simulink model "leuschner_spectrometer"  (Simulink 6.2)
settings: Solver=ode45  StartTime=0.0  StopTime=10  RelTol=1e-3
undefined symbols (not defined in the file): MaxCoeffNum
libraries: xbsIndex_r3 x225, fft_library x17, xps_library x14, delay_lib x4, casper_library x3, simulink x1, pfb_library x1
(part 1 of 2)
settings Model: LastModifiedBy=siemion
settings DebuggingCC: SolverPrmCheckMsg=warning

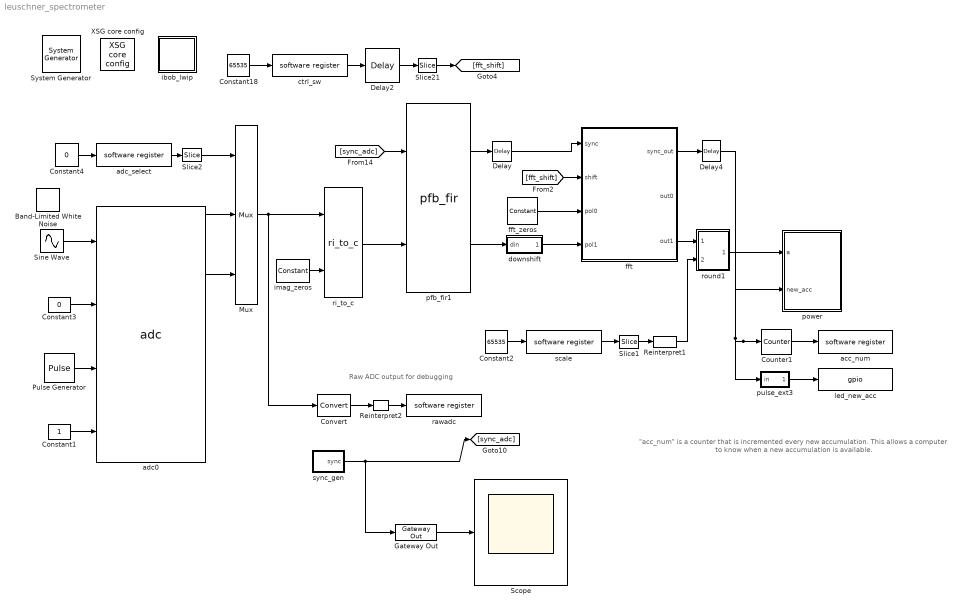
== system leuschner_spectrometer ==
  note: Raw ADC output for debugging
  note: "acc_num" is a counter that is
      | incremented every new accumulation.
      | This allows a computer to know when
      | a new accumulation is available.
  " System Generator" : xbsIndex_r3/ System Generator  Tag=genX  xilinxfamily=Virtex2P  part=xc2vp50  speed=-7  package=ff1152  synthesis_tool=XST  directory=./heilesspec_two_inp/sysgen  testbench=off  simulink_period=1  sysclk_period=41.6667  incr_netlist=off  trim_vbits=Everywhere in SubSystem  dbl_ovrd=According to Block Masks  core_generation=According to Block Masks  run_coregen=off  deprecated_control=off  eval_field=0
      settings: AttributesFormatString=System\nGenerator
  Band-Limited White Noise : simulink/Sources/Band-Limited White Noise  Cov=[0.1]  Ts=0.1  seed=[23341]
  Constant1 : Constant
  Constant18 : Constant  Value=65535
  Constant2 : Constant  Value=65535
  Constant3 : Constant  Value=0
  Constant4 : Constant  Value=0
  Convert : xbsIndex_r3/Convert  arith_type="Signed  (2's comp)"  n_bits=32  bin_pt=7  quantization=Truncate  overflow=Wrap  latency=0  explicit_period=off  period=1  dbl_ovrd=off  show_param=off  inserted_by_tool=off  pipeline=off
      settings: xl_area=[0, 0, 0, 0, 0, 0, 0]
  Counter1 : xbsIndex_r3/Counter  cnt_type=Free Running  n_bits=32  bin_pt=0  arith_type=Unsigned  start_count=0  cnt_to=Inf  cnt_by_val=1  operation=Up  explicit_period=off  period=1  load_pin=off  rst=off  en=on  dbl_ovrd=off  show_param=off  use_rpm=on  gen_core=off
      settings: xl_area=[0, 0, 0, 0, 0, 0, 0]
  Delay : xbsIndex_r3/Delay  latency=2  reg_retiming=off  explicit_period=off  period=1  en=off  accept_only_valid=off  init_zero=on  dbl_ovrd=off  show_param=off
      settings: xl_area=[0, 0, 0, 0, 0, 0, 0]
  Delay2 : xbsIndex_r3/Delay  latency=1  reg_retiming=off  explicit_period=off  period=1  en=off  accept_only_valid=off  init_zero=on  dbl_ovrd=off  show_param=off
      settings: xl_area=[0, 0, 0, 0, 0, 0, 0]
  Delay4 : xbsIndex_r3/Delay  latency=4  reg_retiming=off  explicit_period=off  period=1  en=off  accept_only_valid=off  init_zero=on  dbl_ovrd=off  show_param=off
      settings: xl_area=[0, 0, 0, 0, 0, 0, 0]
  Gateway Out : xbsIndex_r3/Gateway Out  output_type=Double  nbits=8  bin_pt=6  arith_type=Boolean  quantization=Truncate  overflow=Wrap  hdl_port=on  timing_constraint=None  locs_specified=off  LOCs={}  needs_fixed_name=off  show_param=off
      settings: xl_area=[0, 0, 0, 0, 0, 0, 0]
  Mux : xbsIndex_r3/Mux  inputs=2  precision=Full  arith_type="Signed  (2's comp)"  n_bits=8  bin_pt=2  quantization=Truncate  overflow=Wrap  latency=0  explicit_period=off  period=1  en=off  dbl_ovrd=off  show_param=off  mux_type=off  use_rpm=off  gen_core=off
      settings: xl_area=[0, 0, 0, 0, 0, 0, 0]
  Pulse Generator : DiscretePulseGenerator  Period=2^9
  Reinterpret1 : xbsIndex_r3/Reinterpret  force_arith_type=on  arith_type=Unsigned  force_bin_pt=on  bin_pt=3  force_valid=on
  Reinterpret2 : xbsIndex_r3/Reinterpret  force_arith_type=on  arith_type=Unsigned  force_bin_pt=on  bin_pt=0  force_valid=on
  Scope : Scope
      settings: YMin=-1  YMax=1
  Sine Wave : Sin  SineType=Sample based  Amplitude=0.2  Frequency=2*pi*0.5  Samples=8  SampleTime=1
  Slice1 : xbsIndex_r3/Slice  mode=Lower Bit Location + Width  nbits=18  bit1=0  base1=MSB of Input  bit0=0  base0=LSB of Input  boolean_output=off  explicit_period=off  period=1  dbl_ovrd=off
  Slice2 : xbsIndex_r3/Slice  mode=Lower Bit Location + Width  nbits=1  bit1=0  base1=MSB of Input  bit0=0  base0=LSB of Input  boolean_output=on  explicit_period=off  period=1  dbl_ovrd=off
  Slice21 : xbsIndex_r3/Slice  mode=Lower Bit Location + Width  nbits=16  bit1=0  base1=MSB of Input  bit0=0  base0=LSB of Input  boolean_output=off  explicit_period=off  period=1  dbl_ovrd=off
  XSG core config : xps_library/XSG core config  Tag=xps:xsg  hw_sys=iBOB  ibob_linux=off  clk_src=adc0_clk  gpio_clk_io_group=iBOB:sma  gpio_clk_bit_index=0  clk_rate=24  sample_period=1  synthesis_tool=XST  mpc_type=powerpc405
  acc_num : xps_library/software register  Tag=xps:sw_reg  io_dir=To Processor  arith_type=Unsigned  bitwidth=32  bin_pt=0  sample_period=1  gw_name=heilesspec_two_inp_acc_num_user_data_in
  adc0 : xps_library/adc  Tag=xps:adc  adc_brd=iBOB:adc0  adc_clk_rate=96  adc_interleave=off  sample_period=1
  adc_select : xps_library/software register  Tag=xps:sw_reg  io_dir=From Processor  arith_type=Unsigned  bitwidth=32  bin_pt=0  sample_period=1  gw_name=heilesspec_two_inp_adc_select_user_data_out
  ctrl_sw : xps_library/software register  Tag=xps:sw_reg  io_dir=From Processor  arith_type=Unsigned  bitwidth=32  bin_pt=0  sample_period=1  gw_name=heilesspec_two_inp_ctrl_sw_user_data_out
  downshift : Subsystem
  fft : Subsystem  AncestorBlock=fft_library/fft  mask{FFTSize=14, BitWidth=18, n_inputs=0, quantization=Truncate, overflow=Wrap, add_latency=2, mult_latency=4, bram_latency=1}
      mask prompts: FFTSize "Size of FFT: (2^?)"; BitWidth "Bit Width"; n_inputs "Number of Simultaneous Inputs: (2^?)"; quantization "Quantization Behavior"; overflow "Overflow Behavior"; add_latency "Add Latency"; mult_latency "Mult Latency"; bram_latency "BRAM Latency"
      mask init:
      | fft_mask;
      mask StyleString: edit,edit,edit,popup(Truncate|Round  (unbiased: +/- Inf)|Round  (unbiased: Even Values)),popup(Wrap|Saturate|Error),edit,edit,edit
  fft_zeros : xbsIndex_r3/Constant  const=0  equ=P=C  arith_type=Unsigned  n_bits=36  bin_pt=0  opselect=C  inp2=PCIN>>17  opr=+  inp1=P  carry=CIN  iostate=0  explicit_period=on  period=1  dbl_ovrd=off
  ibob_lwip : Subsystem  AncestorBlock=xps_library/ibob_lwip
      mask Type: ibobethlite
      mask Description: Attaches SRAM0 to the PLB bus and adds LWIP support.
      mask Display: fprintf('IBOB\nLWIP');
  imag_zeros : xbsIndex_r3/Constant  const=0  equ=P=C  arith_type="Signed  (2's comp)"  n_bits=8  bin_pt=7  opselect=C  inp2=PCIN>>17  opr=+  inp1=P  carry=CIN  iostate=0  explicit_period=on  period=1  dbl_ovrd=off
  led_new_acc : xps_library/gpio  Tag=xps:gpio  io_group=iBOB:led  io_dir=out  arith_type=Boolean  bitwidth=1  bin_pt=0  bit_index=5  sample_period=1  use_single_ended=off  use_ddr=off  reg_iob=on  reg_clk_phase=0  termination=None
  pfb_fir1 : pfb_library/pfb_fir  PFBSize=14  TotalTaps=2  WindowType=hamming  n_inputs=0  MakeBiplex=off  BitWidthIn=8  BitWidthOut=18  CoeffBitWidth=8  CoeffDistMem=on  add_latency=2  mult_latency=3  bram_latency=2  quantization="Round  (unbiased: +/- Inf)"  fwidth=1
      link override pol1_in1_first_tap/sync_delay/Constant: equ=P=C
      link override pol1_in1_first_tap/sync_delay/Constant1: equ=P=C
      link override pol1_in1_first_tap/sync_delay/Constant2: equ=P=C
      link override pol1_in1_first_tap/sync_delay/Constant3: equ=P=C
  power : Subsystem
  pulse_ext3 : Subsystem  mask{pulse_len=2^23}
      mask prompts: pulse_len "Length of Pulse"
      mask init:
      | bits = ceil(log2(pulse_len+1));
  rawadc : xps_library/software register  Tag=xps:sw_reg  io_dir=To Processor  arith_type=Unsigned  bitwidth=32  bin_pt=0  sample_period=1  gw_name=heilesspec_two_inp_rawadc_user_data_in
  ri_to_c : fft_library/ri_to_c  likes_cookies=on
  round1 : Subsystem
  scale : xps_library/software register  Tag=xps:sw_reg  io_dir=From Processor  arith_type=Unsigned  bitwidth=32  bin_pt=0  sample_period=1  gw_name=heilesspec_two_inp_scale_user_data_out
  sync_gen : Subsystem
  wires:
  Pulse Generator/1 -> adc0/3
  Constant1/1 -> adc0/4
  pfb_fir1/1 -> Delay/1
  sync_gen/1(sync) -> Gateway Out/1, [sync_adc]
  Constant18/1 -> ctrl_sw/1
  ctrl_sw/1 -> Delay2/1
  Slice21/1 -> [fft_shift]
  [sync_adc] -> pfb_fir1/1
  [fft_shift] -> fft/2(shift)
  fft/1(sync_out) -> Delay4/1
  pulse_ext3/1(out) -> led_new_acc/1
  Counter1/1 -> acc_num/1
  Delay2/1 -> Slice21/1
  pfb_fir1/2 -> downshift/1(din)
  Delay/1 -> fft/1(sync)
  Gateway Out/1 -> Scope/1
  Constant3/1 -> adc0/2
  imag_zeros/1 -> ri_to_c/2
  ri_to_c/1 -> pfb_fir1/2
  downshift/1(dout) -> fft/4(pol1)
  Sine Wave/1 -> adc0/1
  fft_zeros/1 -> fft/3(pol0)
  Reinterpret1/1 -> round1/2(scale)
  Delay4/1 -> power/2(new_acc), pulse_ext3/1(in), Counter1/1
  fft/3(out1) -> round1/1(din)
  Constant2/1 -> scale/1
  scale/1 -> Slice1/1
  Slice1/1 -> Reinterpret1/1
  adc0/1 -> Mux/2
  adc0/5 -> Mux/3
  Slice2/1 -> Mux/1
  adc_select/1 -> Slice2/1
  Convert/1 -> Reinterpret2/1
  Mux/1 -> Convert/1, ri_to_c/1
  Reinterpret2/1 -> rawadc/1
  Constant4/1 -> adc_select/1
  round1/1(dout) -> power/1(a)

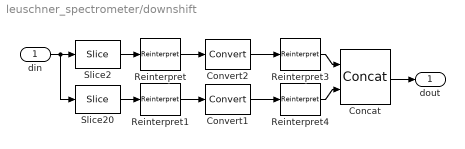
== system leuschner_spectrometer/downshift ==
  din : Inport  Port=1  LatchInput=off
  Concat : xbsIndex_r3/Concat  num_inputs=2  explicit_period=off  period=1  dbl_ovrd=off
  Convert1 : xbsIndex_r3/Convert  arith_type="Signed  (2's comp)"  n_bits=18  bin_pt=15  quantization="Round  (unbiased: Even Values)"  overflow=Wrap  latency=2  explicit_period=off  period=1  dbl_ovrd=off  show_param=off  inserted_by_tool=off  pipeline=off
      settings: xl_area=[0, 0, 0, 0, 0, 0, 0]
  Convert2 : xbsIndex_r3/Convert  arith_type="Signed  (2's comp)"  n_bits=18  bin_pt=15  quantization="Round  (unbiased: Even Values)"  overflow=Wrap  latency=2  explicit_period=off  period=1  dbl_ovrd=off  show_param=off  inserted_by_tool=off  pipeline=off
      settings: xl_area=[0, 0, 0, 0, 0, 0, 0]
  Reinterpret : xbsIndex_r3/Reinterpret  force_arith_type=on  arith_type="Signed  (2's comp)"  force_bin_pt=on  bin_pt=17  force_valid=on
  Reinterpret1 : xbsIndex_r3/Reinterpret  force_arith_type=on  arith_type="Signed  (2's comp)"  force_bin_pt=on  bin_pt=17  force_valid=on
  Reinterpret3 : xbsIndex_r3/Reinterpret  force_arith_type=on  arith_type=Unsigned  force_bin_pt=on  bin_pt=0  force_valid=on
  Reinterpret4 : xbsIndex_r3/Reinterpret  force_arith_type=on  arith_type=Unsigned  force_bin_pt=on  bin_pt=0  force_valid=on
  Slice2 : xbsIndex_r3/Slice  mode=Upper Bit Location + Width  nbits=18  bit1=0  base1=MSB of Input  bit0=0  base0=LSB of Input  boolean_output=off  explicit_period=off  period=1  dbl_ovrd=off
  Slice20 : xbsIndex_r3/Slice  mode=Lower Bit Location + Width  nbits=18  bit1=0  base1=MSB of Input  bit0=0  base0=LSB of Input  boolean_output=off  explicit_period=off  period=1  dbl_ovrd=off
  dout : Outport
  wires:
  Slice2/1 -> Reinterpret/1
  Slice20/1 -> Reinterpret1/1
  din/1 -> Slice2/1, Slice20/1
  Reinterpret3/1 -> Concat/1
  Reinterpret4/1 -> Concat/2
  Concat/1 -> dout/1
  Reinterpret/1 -> Convert2/1
  Reinterpret1/1 -> Convert1/1
  Convert2/1 -> Reinterpret3/1
  Convert1/1 -> Reinterpret4/1

== system leuschner_spectrometer/fft ==
  sync : Inport  Port=1  LatchInput=off
  shift : Inport  Port=2  LatchInput=off
  pol0 : Inport  Port=3  LatchInput=off
  pol1 : Inport  Port=4  LatchInput=off
  fft_biplex0 : Subsystem  AncestorBlock=fft_library/fft_biplex  mask(fft_biplex){FFTSize=FFTSize-n_inputs, BitWidth=BitWidth, quantization=Truncate, overflow=Wrap, add_latency=add_latency, mult_latency=mult_latency, bram_latency=bram_latency}
      mask prompts: FFTSize "Size of FFT: (2^? pnts)"; BitWidth "Bitwidth: (Max Efficiency at 18 bits)"; quantization "Quantization Behavior"; overflow "Overflow Behavior"; add_latency "Add Latency"; mult_latency "Mult Latency"; bram_latency "BRAM Latency"
      mask init:
      | cursys = gcb;
      | disp(cursys);
      | biplex_core = [cursys,'/biplex_core'];
      | if ~strcmp(get_param(biplex_core, 'quantization'), quantization),
      |     set_param(biplex_core, 'quantization', quantization);
      | end
      | if ~strcmp(get_param(biplex_core, 'overflow'), overflow),
      |     set_param(biplex_core, 'overflow', overflow);
      | end
      mask StyleString: edit,edit,popup(Truncate|Round  (unbiased: +/- Inf)|Round  (unbiased: Even Values)),popup(Wrap|Saturate|Error),edit,edit,edit
  sync_out : Outport
  out0 : Outport  Port=2
  out1 : Outport  Port=3

== system leuschner_spectrometer/ibob_lwip ==
  Constant : Constant  Value=0
  Terminator : Terminator
  ethlite : Subsystem  Tag=xps:ethlite
      mask Type: ethlite
      mask Description: Instantiates an opb_ethernetlite core into the design.
      mask Display: fprintf('ETHLITE');
  lwip : Subsystem  Tag=xps:lwip
      mask Type: lwip
      mask Description: Attaches SRAM0 to the PLB bus and adds LWIP support.
      mask Display: fprintf('LWIP');
  macbits : xps_library/software register  Tag=xps:sw_reg  io_dir=To Processor  arith_type=Unsigned  bitwidth=32  bin_pt=0  sample_period=1  gw_name=heilesspec_two_inp_ibob_lwip_macbits_user_data_in
  machdr : xps_library/gpio  Tag=xps:gpio  io_group=iBOB:gpio2  io_dir=in  arith_type=Unsigned  bitwidth=20  bin_pt=0  bit_index=[0:19]  sample_period=1  use_single_ended=off  use_ddr=off  reg_iob=off  reg_clk_phase=0  termination=Pullup
  wires:
  Constant/1 -> machdr/1
  macbits/1 -> Terminator/1
  machdr/1 -> macbits/1

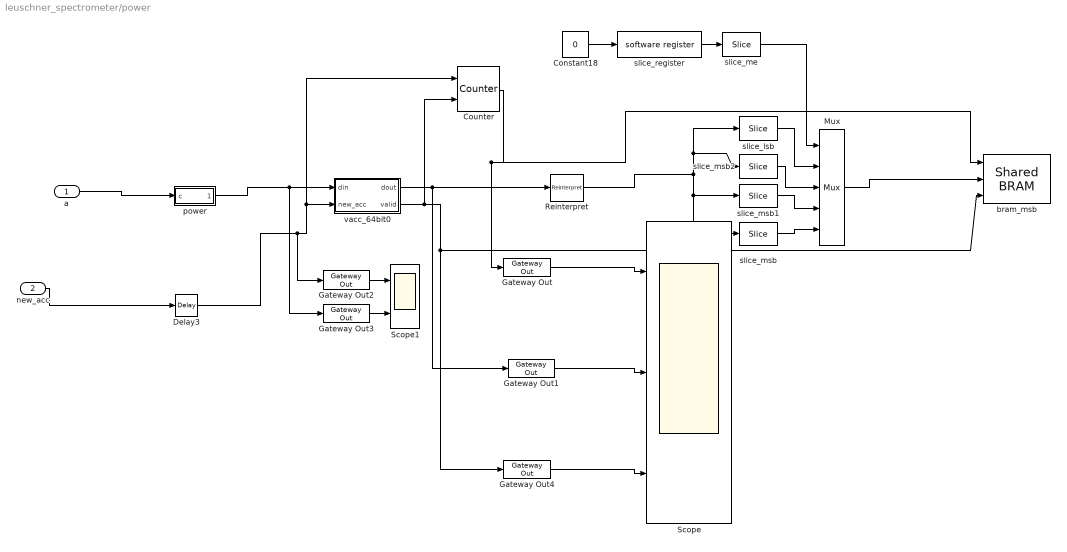
== system leuschner_spectrometer/power ==
  a : Inport  Port=1  LatchInput=off
  new_acc : Inport  Port=2  LatchInput=off
  Constant18 : Constant  Value=0
  Counter : xbsIndex_r3/Counter  cnt_type=Free Running  n_bits=13  bin_pt=0  arith_type=Unsigned  start_count=0  cnt_to=Inf  cnt_by_val=1  operation=Up  explicit_period=off  period=1  load_pin=off  rst=on  en=on  dbl_ovrd=off  show_param=off  use_rpm=on  gen_core=off
      settings: xl_area=[0, 0, 0, 0, 0, 0, 0]
  Delay3 : xbsIndex_r3/Delay  latency=5  reg_retiming=off  explicit_period=off  period=1  en=off  accept_only_valid=off  init_zero=on  dbl_ovrd=off  show_param=off
      settings: xl_area=[0, 0, 0, 0, 0, 0, 0]
  Gateway Out{,1..4} (5 alike) : xbsIndex_r3/Gateway Out  output_type=Double  nbits=8  bin_pt=6  arith_type=Boolean  quantization=Truncate  overflow=Wrap  hdl_port=on  timing_constraint=None  locs_specified=off  LOCs={}  needs_fixed_name=off  show_param=off
      settings: xl_area=[0, 0, 0, 0, 0, 0, 0]
  Mux : xbsIndex_r3/Mux  inputs=4  precision=Full  arith_type="Signed  (2's comp)"  n_bits=8  bin_pt=2  quantization=Truncate  overflow=Wrap  latency=0  explicit_period=off  period=1  en=off  dbl_ovrd=off  show_param=off  mux_type=off  use_rpm=off  gen_core=off
      settings: xl_area=[0, 0, 0, 0, 0, 0, 0]
  Reinterpret : xbsIndex_r3/Reinterpret  force_arith_type=on  arith_type="Signed  (2's comp)"  force_bin_pt=on  bin_pt=0  force_valid=on
  Scope : Scope  NumInputPorts=3
      settings: YMin=0~0~0  YMax=2100~0.00095~1
  Scope1 : Scope  NumInputPorts=2
      settings: YMin=-1~0  YMax=1~0.00045  SaveName=ScopeData2
  bram_msb : xps_library/Shared BRAM  Tag=xps:bram  arith_type=Unsigned  addr_width=13  data_width=32  data_bin_pt=0  init_vals=[1:2^11]  sample_rate=1
  power : Subsystem  AncestorBlock=casper_library/Misc/power  mask{BitWidth=18}
      mask prompts: BitWidth "Bit Width"
  slice_lsb : xbsIndex_r3/Slice  mode=Lower Bit Location + Width  nbits=32  bit1=0  base1=LSB of Input  bit0=0  base0=LSB of Input  boolean_output=off  explicit_period=off  period=1  dbl_ovrd=off
  slice_me : xbsIndex_r3/Slice  mode=Lower Bit Location + Width  nbits=2  bit1=0  base1=LSB of Input  bit0=0  base0=LSB of Input  boolean_output=off  explicit_period=off  period=1  dbl_ovrd=off
  slice_msb : xbsIndex_r3/Slice  mode=Lower Bit Location + Width  nbits=32  bit1=0  base1=LSB of Input  bit0=32  base0=LSB of Input  boolean_output=off  explicit_period=off  period=1  dbl_ovrd=off
  slice_msb1 : xbsIndex_r3/Slice  mode=Lower Bit Location + Width  nbits=32  bit1=0  base1=LSB of Input  bit0=16  base0=LSB of Input  boolean_output=off  explicit_period=off  period=1  dbl_ovrd=off
  slice_msb2 : xbsIndex_r3/Slice  mode=Lower Bit Location + Width  nbits=32  bit1=0  base1=LSB of Input  bit0=8  base0=LSB of Input  boolean_output=off  explicit_period=off  period=1  dbl_ovrd=off
  slice_register : xps_library/software register  Tag=xps:sw_reg  io_dir=From Processor  arith_type=Unsigned  bitwidth=32  bin_pt=0  sample_period=1  gw_name=heilesspec_two_inp_power_slice_register_user_data_out
  vacc_64bit0 : Subsystem
  wires:
  new_acc/1 -> Delay3/1
  power/1(power) -> vacc_64bit0/1(din), Gateway Out3/1
  vacc_64bit0/1(dout) -> Reinterpret/1, Gateway Out1/1
  Delay3/1 -> Counter/1, vacc_64bit0/2(new_acc), Gateway Out2/1
  vacc_64bit0/2(valid) -> Counter/2, bram_msb/3, Gateway Out4/1
  Counter/1 -> Gateway Out/1, bram_msb/1
  Gateway Out/1 -> Scope/1
  Gateway Out1/1 -> Scope/2
  Gateway Out2/1 -> Scope1/1
  Gateway Out3/1 -> Scope1/2
  a/1 -> power/1(c)
  Reinterpret/1 -> slice_lsb/1, slice_msb2/1, slice_msb/1, slice_msb1/1
  Gateway Out4/1 -> Scope/3
  slice_lsb/1 -> Mux/2
  Mux/1 -> bram_msb/2
  slice_register/1 -> slice_me/1
  Constant18/1 -> slice_register/1
  slice_me/1 -> Mux/1
  slice_msb2/1 -> Mux/3
  slice_msb1/1 -> Mux/4
  slice_msb/1 -> Mux/5

== system leuschner_spectrometer/pulse_ext3 ==
  in : Inport  Port=1  LatchInput=off
  Constant5 : xbsIndex_r3/Constant  const=pulse_len  equ=P=C  arith_type=Unsigned  n_bits=bits  bin_pt=0  opselect=C  inp2=PCIN>>17  opr=+  inp1=P  carry=CIN  iostate=0  explicit_period=off  period=1  dbl_ovrd=off
  Counter3 : xbsIndex_r3/Counter  cnt_type=Free Running  n_bits=bits  bin_pt=0  arith_type=Unsigned  start_count=0  cnt_to=1023  cnt_by_val=1  operation=Up  explicit_period=on  period=1  load_pin=off  rst=on  en=on  dbl_ovrd=off  show_param=off  use_rpm=on  gen_core=off
      settings: xl_area=[0, 0, 0, 0, 0, 0, 0]
  Relational5 : xbsIndex_r3/Relational  mode=a!=b  latency=0  explicit_period=off  period=1  en=off  dbl_ovrd=off  show_param=off
      settings: xl_area=[0, 0, 0, 0, 0, 0, 0]
  posedge : Subsystem  Tag=Rising Edge Detector
  out : Outport
  wires:
  Counter3/1 -> Relational5/1
  Constant5/1 -> Relational5/2
  Relational5/1 -> Counter3/2, out/1
  in/1 -> posedge/1(In)
  posedge/1(Out) -> Counter3/1

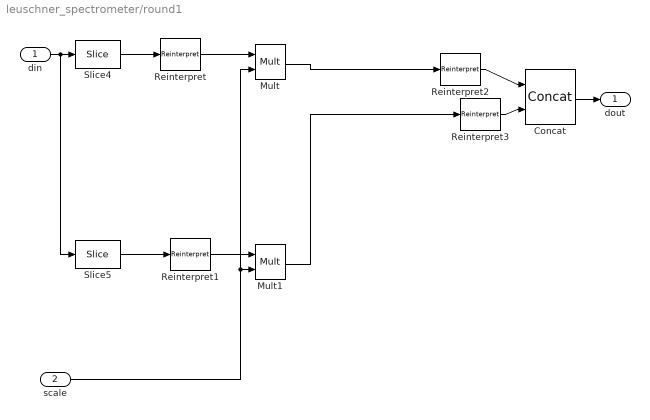
== system leuschner_spectrometer/round1 ==
  din : Inport  Port=1  LatchInput=off
  scale : Inport  Port=2  LatchInput=off
  Concat : xbsIndex_r3/Concat  num_inputs=2  explicit_period=off  period=1  dbl_ovrd=off
  Mult : xbsIndex_r3/Mult  precision=User Defined  arith_type="Signed  (2's comp)"  n_bits=18  bin_pt=17  quantization=Truncate  overflow=Saturate  latency=4  explicit_period=off  period=1  en=off  dbl_ovrd=off  show_param=on  mult_type=Parallel  oversample=2  use_embedded=on  pipeline=on  use_rpm=on  placement_style=Rectangular Shape  gen_core=off
      settings: xl_area=[0, 0, 0, 0, 0, 0, 0]
  Mult1 : xbsIndex_r3/Mult  precision=User Defined  arith_type="Signed  (2's comp)"  n_bits=18  bin_pt=17  quantization=Truncate  overflow=Saturate  latency=4  explicit_period=off  period=1  en=off  dbl_ovrd=off  show_param=on  mult_type=Parallel  oversample=2  use_embedded=on  pipeline=on  use_rpm=on  placement_style=Rectangular Shape  gen_core=off
      settings: xl_area=[0, 0, 0, 0, 0, 0, 0]
  Reinterpret : xbsIndex_r3/Reinterpret  force_arith_type=on  arith_type="Signed  (2's comp)"  force_bin_pt=on  bin_pt=17  force_valid=on
  Reinterpret1 : xbsIndex_r3/Reinterpret  force_arith_type=on  arith_type="Signed  (2's comp)"  force_bin_pt=on  bin_pt=17  force_valid=on
  Reinterpret2 : xbsIndex_r3/Reinterpret  force_arith_type=on  arith_type=Unsigned  force_bin_pt=on  bin_pt=0  force_valid=on
  Reinterpret3 : xbsIndex_r3/Reinterpret  force_arith_type=on  arith_type=Unsigned  force_bin_pt=on  bin_pt=0  force_valid=on
  Slice4 : xbsIndex_r3/Slice  mode=Upper Bit Location + Width  nbits=18  bit1=0  base1=MSB of Input  bit0=0  base0=LSB of Input  boolean_output=off  explicit_period=off  period=1  dbl_ovrd=off
  Slice5 : xbsIndex_r3/Slice  mode=Lower Bit Location + Width  nbits=18  bit1=0  base1=MSB of Input  bit0=0  base0=LSB of Input  boolean_output=off  explicit_period=off  period=1  dbl_ovrd=off
  dout : Outport
  wires:
  Slice4/1 -> Reinterpret/1
  Reinterpret2/1 -> Concat/1
  Slice5/1 -> Reinterpret1/1
  Reinterpret3/1 -> Concat/2
  din/1 -> Slice4/1, Slice5/1
  Concat/1 -> dout/1
  Reinterpret1/1 -> Mult1/1
  Reinterpret/1 -> Mult/1
  scale/1 -> Mult1/2, Mult/2
  Mult/1 -> Reinterpret2/1
  Mult1/1 -> Reinterpret3/1

== system leuschner_spectrometer/sync_gen ==
  note: NOTE: Outputs sync pulse immediately on RST
      | (i.e. when RST goes high, SYNC goes high, and the sync counter is reset)
  note: PERIOD must be the period you want, sub 2.
      | e.g. If you want 2048, enter 2046
  Constant : Constant  Value=2^12 * 8
  Convert : xbsIndex_r3/Convert  arith_type=Boolean  n_bits=8  bin_pt=6  quantization=Truncate  overflow=Wrap  latency=1  explicit_period=off  period=1  dbl_ovrd=off  show_param=off  inserted_by_tool=off  pipeline=off
      settings: xl_area=[0, 0, 0, 0, 0, 0, 0]
  Counter1 : xbsIndex_r3/Counter  cnt_type=Free Running  n_bits=32  bin_pt=0  arith_type=Unsigned  start_count=1  cnt_to=Inf  cnt_by_val=1  operation=Up  explicit_period=on  period=1  load_pin=off  rst=on  en=off  dbl_ovrd=off  show_param=off  use_rpm=on  gen_core=off
      settings: xl_area=[0, 0, 0, 0, 0, 0, 0]
  Relational : xbsIndex_r3/Relational  mode=a>=b  latency=1  explicit_period=off  period=1  en=off  dbl_ovrd=off  show_param=off
      settings: xl_area=[0, 0, 0, 0, 0, 0, 0]
  period : xps_library/software register  Tag=xps:sw_reg  io_dir=From Processor  arith_type=Unsigned  bitwidth=32  bin_pt=0  sample_period=1  gw_name=heilesspec_two_inp_sync_gen_period_user_data_out
  sync : Outport
  wires:
  Counter1/1 -> Relational/1
  Relational/1 -> Convert/1
  period/1 -> Relational/2
  Convert/1 -> Counter1/1, sync/1
  Constant/1 -> period/1

== system leuschner_spectrometer/fft/fft_biplex0 ==
  pol1 : Inport  Port=1  LatchInput=off
  pol2 : Inport  Port=2  LatchInput=off
  sync : Inport  Port=3  LatchInput=off
  shift : Inport  Port=4  LatchInput=off
  biplex_core : Subsystem  AncestorBlock=fft_library/biplex_core  mask{FFTSize=FFTSize, BitWidth=BitWidth, quantization=Truncate, overflow=Wrap, add_latency=add_latency, mult_latency=mult_latency, bram_latency=bram_latency}
      mask prompts: FFTSize "Size of FFT: (2^? pnts)"; BitWidth "Bitwidth: (Max Efficiency at 18 bits)"; quantization "Quantization Behavior"; overflow "Overflow Behavior"; add_latency "Add Latency"; mult_latency "Mult Latency"; bram_latency "BRAM Latency"
      mask init:
      | biplex_core_mask;
      mask StyleString: edit,edit,popup(Truncate|Round  (unbiased: +/- Inf)|Round  (unbiased: Even Values)),popup(Wrap|Saturate|Error),edit,edit,edit
  biplex_cplx_unscrambler : Subsystem
  pol1_out : Outport
  pol2_out : Outport  Port=2
  of : Outport  Port=3
  sync_out : Outport  Port=4
  wires:
  biplex_core/4(sync_out) -> biplex_cplx_unscrambler/3(sync)
  biplex_core/2(out2) -> biplex_cplx_unscrambler/2(odd)
  biplex_core/1(out1) -> biplex_cplx_unscrambler/1(even)
  biplex_core/3(of) -> of/1
  biplex_cplx_unscrambler/3(sync_out) -> sync_out/1
  biplex_cplx_unscrambler/2(pol2) -> pol2_out/1
  biplex_cplx_unscrambler/1(pol1) -> pol1_out/1
  shift/1 -> biplex_core/4(shift)
  sync/1 -> biplex_core/3(sync)
  pol2/1 -> biplex_core/2(pol2)
  pol1/1 -> biplex_core/1(pol1)

== system leuschner_spectrometer/ibob_lwip/ethlite ==

== system leuschner_spectrometer/ibob_lwip/lwip ==

== system leuschner_spectrometer/power/power ==
  c : Inport  Port=1  LatchInput=off
  c_to_ri : casper_library/Misc/c_to_ri  n_bits=BitWidth  bin_pt=BitWidth-1
      settings: AttributesFormatString=18_17 r/i
  imag_square : xbsIndex_r3/Mult  precision=Full  arith_type="Signed  (2's comp)"  n_bits=8  bin_pt=2  quantization=Truncate  overflow=Wrap  latency=3  explicit_period=off  period=1  en=off  dbl_ovrd=off  show_param=on  mult_type=Parallel  oversample=2  use_embedded=on  pipeline=on  use_rpm=on  placement_style=Rectangular Shape  gen_core=off
      settings: xl_area=[0, 0, 0, 0, 0, 0, 0]
  power_adder : xbsIndex_r3/AddSub  mode=Addition  precision=User Defined  arith_type=Unsigned  n_bits=BitWidth * 2  bin_pt=BitWidth * 2 - 1  quantization=Truncate  overflow=Wrap  latency=2  explicit_period=off  period=1  use_carryin=off  use_carryout=off  en=off  dbl_ovrd=off  show_param=off  use_core=on  pipeline=off  use_rpm=on  gen_core=off
      settings: xl_area=[0, 0, 0, 0, 0, 0, 0]
  real_square : xbsIndex_r3/Mult  precision=Full  arith_type="Signed  (2's comp)"  n_bits=8  bin_pt=2  quantization=Truncate  overflow=Wrap  latency=3  explicit_period=off  period=1  en=off  dbl_ovrd=off  show_param=on  mult_type=Parallel  oversample=2  use_embedded=on  pipeline=on  use_rpm=on  placement_style=Rectangular Shape  gen_core=off
      settings: xl_area=[0, 0, 0, 0, 0, 0, 0]
  power : Outport
  wires:
  power_adder/1 -> power/1
  imag_square/1 -> power_adder/2
  real_square/1 -> power_adder/1
  c/1 -> c_to_ri/1
  c_to_ri/1 -> real_square/1, real_square/2
  c_to_ri/2 -> imag_square/2, imag_square/1

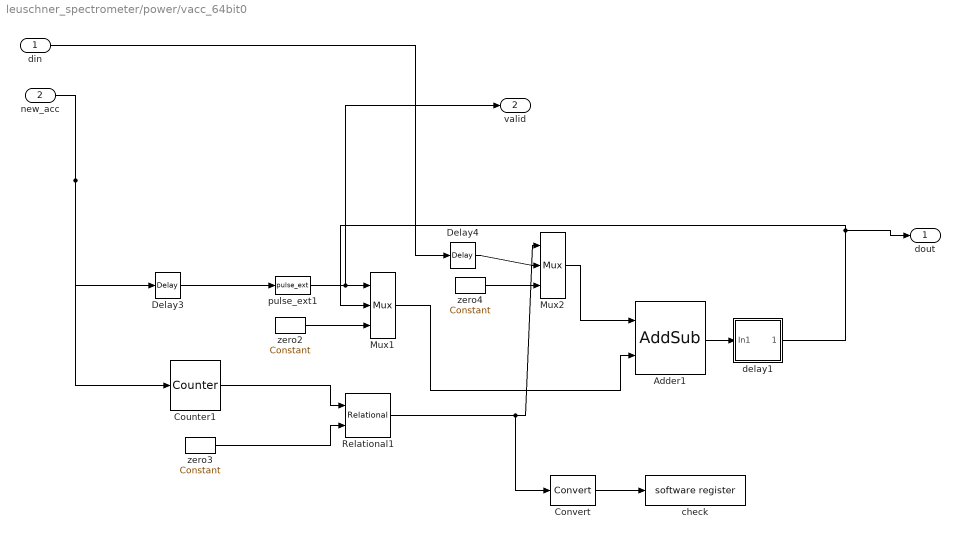
== system leuschner_spectrometer/power/vacc_64bit0 ==
  din : Inport  Port=1  LatchInput=off
  new_acc : Inport  Port=2  LatchInput=off
  Adder1 : xbsIndex_r3/AddSub  mode=Addition  precision=User Defined  arith_type=Unsigned  n_bits=64  bin_pt=35  quantization=Truncate  overflow=Wrap  latency=4  explicit_period=on  period=1  use_carryin=off  use_carryout=off  en=off  dbl_ovrd=off  show_param=on  use_core=on  pipeline=on  use_rpm=on  gen_core=off
      settings: xl_area=[0, 0, 0, 0, 0, 0, 0]
  Convert : xbsIndex_r3/Convert  arith_type=Unsigned  n_bits=32  bin_pt=0  quantization=Truncate  overflow=Wrap  latency=0  explicit_period=off  period=1  dbl_ovrd=off  show_param=off  inserted_by_tool=off  pipeline=off
      settings: xl_area=[0, 0, 0, 0, 0, 0, 0]
  Counter1 : xbsIndex_r3/Counter  cnt_type=Free Running  n_bits=14  bin_pt=0  arith_type=Unsigned  start_count=0  cnt_to=Inf  cnt_by_val=1  operation=Up  explicit_period=off  period=1  load_pin=off  rst=on  en=off  dbl_ovrd=off  show_param=off  use_rpm=on  gen_core=off
      settings: xl_area=[0, 0, 0, 0, 0, 0, 0]
  Delay3 : xbsIndex_r3/Delay  latency=1  reg_retiming=off  explicit_period=off  period=1  en=off  accept_only_valid=off  init_zero=on  dbl_ovrd=off  show_param=off
      settings: xl_area=[0, 0, 0, 0, 0, 0, 0]
  Delay4 : xbsIndex_r3/Delay  latency=2  reg_retiming=off  explicit_period=off  period=1  en=off  accept_only_valid=off  init_zero=on  dbl_ovrd=off  show_param=off
      settings: xl_area=[0, 0, 0, 0, 0, 0, 0]
  Mux1 : xbsIndex_r3/Mux  inputs=2  precision=Full  arith_type="Signed  (2's comp)"  n_bits=8  bin_pt=2  quantization=Truncate  overflow=Wrap  latency=0  explicit_period=off  period=1  en=off  dbl_ovrd=off  show_param=off  mux_type=off  use_rpm=off  gen_core=off
      settings: xl_area=[0, 0, 0, 0, 0, 0, 0]
  Mux2 : xbsIndex_r3/Mux  inputs=2  precision=Full  arith_type="Signed  (2's comp)"  n_bits=8  bin_pt=2  quantization=Truncate  overflow=Wrap  latency=0  explicit_period=off  period=1  en=off  dbl_ovrd=off  show_param=off  mux_type=off  use_rpm=off  gen_core=off
      settings: xl_area=[0, 0, 0, 0, 0, 0, 0]
  Relational1 : xbsIndex_r3/Relational  mode=a>=b  latency=1  explicit_period=off  period=1  en=off  dbl_ovrd=off  show_param=off
      settings: xl_area=[0, 0, 0, 0, 0, 0, 0]
  check : xps_library/software register  Tag=xps:sw_reg  io_dir=To Processor  arith_type=Unsigned  bitwidth=32  bin_pt=0  sample_period=1  gw_name=heilesspec_two_inp_power_vacc_64bit0_check_user_data_in
  delay1 : Subsystem  BlockChoice=delay_bram
      link override delay_bram: DelayLen=2^13-4  bram_latency=2
      link override delay_bram/Constant2: equ=P=C
      settings: AttributesFormatString=%<BlockChoice>  TemplateBlock=casper_library/Delays/delay  MemberBlocks=delay_bram,delay_slr
  pulse_ext1 : casper_library/Misc/pulse_ext  pulse_len=2^13
  zero2 : xbsIndex_r3/Constant  const=0  equ=P=C  arith_type=Unsigned  n_bits=64  bin_pt=35  opselect=C  inp2=PCIN>>17  opr=+  inp1=P  carry=CIN  iostate=0  explicit_period=on  period=1  dbl_ovrd=off
  zero3 : xbsIndex_r3/Constant  const=2^13  equ=P=C  arith_type=Unsigned  n_bits=14  bin_pt=0  opselect=C  inp2=PCIN>>17  opr=+  inp1=P  carry=CIN  iostate=0  explicit_period=on  period=1  dbl_ovrd=off
  zero4 : xbsIndex_r3/Constant  const=0  equ=P=C  arith_type=Unsigned  n_bits=36  bin_pt=35  opselect=C  inp2=PCIN>>17  opr=+  inp1=P  carry=CIN  iostate=0  explicit_period=on  period=1  dbl_ovrd=off
  dout : Outport
  valid : Outport  Port=2
  wires:
  Adder1/1 -> delay1/1(In1)
  pulse_ext1/1 -> Mux1/1, valid/1
  Mux1/1 -> Adder1/2
  zero2/1 -> Mux1/3
  zero3/1 -> Relational1/2
  Counter1/1 -> Relational1/1
  Delay3/1 -> pulse_ext1/1
  Relational1/1 -> Mux2/1, Convert/1
  delay1/1(Out1) -> Mux1/2, dout/1
  din/1 -> Delay4/1
  new_acc/1 -> Delay3/1, Counter1/1
  Delay4/1 -> Mux2/2
  zero4/1 -> Mux2/3
  Mux2/1 -> Adder1/1
  Convert/1 -> check/1

== system leuschner_spectrometer/pulse_ext3/posedge ==
  In : Inport  Port=1  LatchInput=off
  Delay : xbsIndex_r3/Delay  latency=1  reg_retiming=off  explicit_period=off  period=1  en=off  accept_only_valid=off  init_zero=on  dbl_ovrd=off  show_param=off
      settings: xl_area=[0, 0, 0, 0, 0, 0, 0]
  Inverter : xbsIndex_r3/Inverter  latency=0  explicit_period=off  period=1  en=off  dbl_ovrd=off  show_param=off
      settings: xl_area=[0, 0, 0, 0, 0, 0, 0]
  Logical : xbsIndex_r3/Logical  logical_function=AND  inputs=2  precision=Full  arith_type=Unsigned  n_bits=8  bin_pt=2  align_bp=on  latency=0  explicit_period=off  period=1  en=off  dbl_ovrd=off  show_param=off
      settings: xl_area=[0, 0, 0, 0, 0, 0, 0]
  Out : Outport
  wires:
  Delay/1 -> Inverter/1
  Inverter/1 -> Logical/1
  In/1 -> Delay/1, Logical/2
  Logical/1 -> Out/1

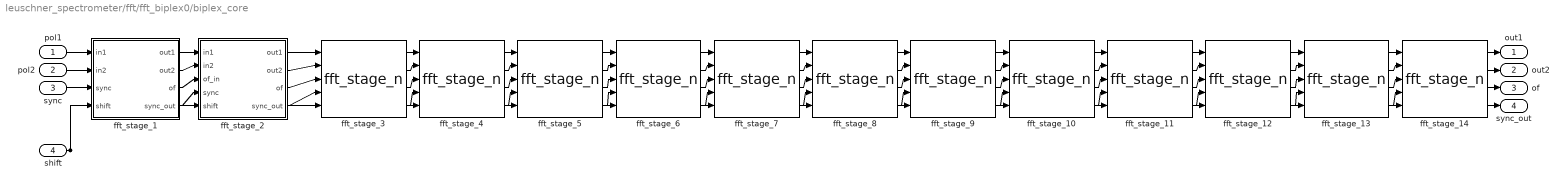
== system leuschner_spectrometer/fft/fft_biplex0/biplex_core ==
  pol1 : Inport  Port=1  LatchInput=off
  pol2 : Inport  Port=2  LatchInput=off
  sync : Inport  Port=3  LatchInput=off
  shift : Inport  Port=4  LatchInput=off
  fft_stage_1 : Subsystem  mask(fft_stage){FFTSize=FFTSize, FFTStage=1, BitWidth=BitWidth, DelayBram=on, CoeffBram=off, MaxCoeffNum=MaxCoeffNum, quantization=Truncate, overflow=Wrap, add_latency=add_latency, mult_latency=mult_latency, bram_latency=bram_latency}
      mask prompts: FFTSize "Size of FFT: (2^? pnts)"; FFTStage "Stage of FFT:"; BitWidth "Output Bitwidth:"; DelayBram "Implement Delays in BRAM:"; CoeffBram "Store Coefficients in BRAM:"; MaxCoeffNum "Maximum Coefficient Depth: (2^?)"; quantization "Quantization Behavior"; overflow "Overflow Behavior"; add_latency "Add Latency"; mult_latency "Mult Latency"; bram_latency "BRAM Latency"
      mask init:
      | fft_stage_n_mask;
      mask StyleString: edit,edit,edit,checkbox,checkbox,edit,popup(Truncate|Round  (unbiased: +/- Inf)|Round  (unbiased: Even Values)),popup(Wrap|Saturate|Error),edit,edit,edit
  fft_stage_10 : fft_library/fft_stage_n  FFTSize=FFTSize  FFTStage=10  BitWidth=BitWidth  DelayBram=off  CoeffBram=on  MaxCoeffNum=MaxCoeffNum  quantization=Truncate  overflow=Wrap  add_latency=add_latency  mult_latency=mult_latency  bram_latency=bram_latency
      link override sync_delay_x/Constant: equ=P=C
      link override sync_delay_x/Constant1: equ=P=C
      link override sync_delay_x/Constant2: equ=P=C
      link override sync_delay_x/Constant3: equ=P=C
  fft_stage_11 : fft_library/fft_stage_n  FFTSize=FFTSize  FFTStage=11  BitWidth=BitWidth  DelayBram=off  CoeffBram=on  MaxCoeffNum=MaxCoeffNum  quantization=Truncate  overflow=Wrap  add_latency=add_latency  mult_latency=mult_latency  bram_latency=bram_latency
      link override sync_delay_x/Constant: equ=P=C
      link override sync_delay_x/Constant1: equ=P=C
      link override sync_delay_x/Constant2: equ=P=C
      link override sync_delay_x/Constant3: equ=P=C
  fft_stage_12 : fft_library/fft_stage_n  FFTSize=FFTSize  FFTStage=12  BitWidth=BitWidth  DelayBram=off  CoeffBram=on  MaxCoeffNum=MaxCoeffNum  quantization=Truncate  overflow=Wrap  add_latency=add_latency  mult_latency=mult_latency  bram_latency=bram_latency
      link override sync_delay_x/Constant: equ=P=C
      link override sync_delay_x/Constant1: equ=P=C
      link override sync_delay_x/Constant2: equ=P=C
      link override sync_delay_x/Constant3: equ=P=C
  fft_stage_13 : fft_library/fft_stage_n  FFTSize=FFTSize  FFTStage=13  BitWidth=BitWidth  DelayBram=off  CoeffBram=on  MaxCoeffNum=MaxCoeffNum  quantization=Truncate  overflow=Wrap  add_latency=add_latency  mult_latency=mult_latency  bram_latency=bram_latency
  fft_stage_14 : fft_library/fft_stage_n  FFTSize=FFTSize  FFTStage=14  BitWidth=BitWidth  DelayBram=off  CoeffBram=on  MaxCoeffNum=MaxCoeffNum  quantization=Truncate  overflow=Wrap  add_latency=add_latency  mult_latency=mult_latency  bram_latency=bram_latency
  fft_stage_2 : Subsystem  mask(fft_stage){FFTSize=FFTSize, FFTStage=2, BitWidth=BitWidth, DelayBram=on, CoeffBram=off, MaxCoeffNum=MaxCoeffNum, quantization=Truncate, overflow=Wrap, add_latency=add_latency, mult_latency=mult_latency, bram_latency=bram_latency}
      mask prompts: FFTSize "Size of FFT: (2^? pnts)"; FFTStage "Stage of FFT:"; BitWidth "Output Bitwidth:"; DelayBram "Implement Delays in BRAM:"; CoeffBram "Store Coefficients in BRAM:"; MaxCoeffNum "Maximum Coefficient Depth: (2^?)"; quantization "Quantization Behavior"; overflow "Overflow Behavior"; add_latency "Add Latency"; mult_latency "Mult Latency"; bram_latency "BRAM Latency"
      mask init:
      | fft_stage_n_mask;
      mask StyleString: edit,edit,edit,checkbox,checkbox,edit,popup(Truncate|Round  (unbiased: +/- Inf)|Round  (unbiased: Even Values)),popup(Wrap|Saturate|Error),edit,edit,edit
  fft_stage_3 : fft_library/fft_stage_n  FFTSize=FFTSize  FFTStage=3  BitWidth=BitWidth  DelayBram=on  CoeffBram=off  MaxCoeffNum=MaxCoeffNum  quantization=Truncate  overflow=Wrap  add_latency=add_latency  mult_latency=mult_latency  bram_latency=bram_latency
      link override delay_b/delay_bram/Constant2: equ=P=C
      link override delay_f/delay_bram/Constant2: equ=P=C
      link override sync_delay_x/Constant: equ=P=C
      link override sync_delay_x/Constant1: equ=P=C
      link override sync_delay_x/Constant2: equ=P=C
      link override sync_delay_x/Constant3: equ=P=C
  fft_stage_4 : fft_library/fft_stage_n  FFTSize=FFTSize  FFTStage=4  BitWidth=BitWidth  DelayBram=on  CoeffBram=off  MaxCoeffNum=MaxCoeffNum  quantization=Truncate  overflow=Wrap  add_latency=add_latency  mult_latency=mult_latency  bram_latency=bram_latency
      link override delay_b/delay_bram/Constant2: equ=P=C
      link override delay_f/delay_bram/Constant2: equ=P=C
      link override sync_delay_x/Constant: equ=P=C
      link override sync_delay_x/Constant1: equ=P=C
      link override sync_delay_x/Constant2: equ=P=C
      link override sync_delay_x/Constant3: equ=P=C
  fft_stage_5 : fft_library/fft_stage_n  FFTSize=FFTSize  FFTStage=5  BitWidth=BitWidth  DelayBram=on  CoeffBram=off  MaxCoeffNum=MaxCoeffNum  quantization=Truncate  overflow=Wrap  add_latency=add_latency  mult_latency=mult_latency  bram_latency=bram_latency
      link override delay_b/delay_bram/Constant2: equ=P=C
      link override delay_f/delay_bram/Constant2: equ=P=C
      link override sync_delay_x/Constant: equ=P=C
      link override sync_delay_x/Constant1: equ=P=C
      link override sync_delay_x/Constant2: equ=P=C
      link override sync_delay_x/Constant3: equ=P=C
  fft_stage_6 : fft_library/fft_stage_n  FFTSize=FFTSize  FFTStage=6  BitWidth=BitWidth  DelayBram=on  CoeffBram=off  MaxCoeffNum=MaxCoeffNum  quantization=Truncate  overflow=Wrap  add_latency=add_latency  mult_latency=mult_latency  bram_latency=bram_latency
      link override delay_b/delay_bram/Constant2: equ=P=C
      link override delay_f/delay_bram/Constant2: equ=P=C
      link override sync_delay_x/Constant: equ=P=C
      link override sync_delay_x/Constant1: equ=P=C
      link override sync_delay_x/Constant2: equ=P=C
      link override sync_delay_x/Constant3: equ=P=C
  fft_stage_7 : fft_library/fft_stage_n  FFTSize=FFTSize  FFTStage=7  BitWidth=BitWidth  DelayBram=on  CoeffBram=off  MaxCoeffNum=MaxCoeffNum  quantization=Truncate  overflow=Wrap  add_latency=add_latency  mult_latency=mult_latency  bram_latency=bram_latency
      link override delay_b/delay_bram/Constant2: equ=P=C
      link override delay_f/delay_bram/Constant2: equ=P=C
      link override sync_delay_x/Constant: equ=P=C
      link override sync_delay_x/Constant1: equ=P=C
      link override sync_delay_x/Constant2: equ=P=C
      link override sync_delay_x/Constant3: equ=P=C
  fft_stage_8 : fft_library/fft_stage_n  FFTSize=FFTSize  FFTStage=8  BitWidth=BitWidth  DelayBram=on  CoeffBram=on  MaxCoeffNum=MaxCoeffNum  quantization=Truncate  overflow=Wrap  add_latency=add_latency  mult_latency=mult_latency  bram_latency=bram_latency
      link override sync_delay_x/Constant: equ=P=C
      link override sync_delay_x/Constant1: equ=P=C
      link override sync_delay_x/Constant2: equ=P=C
      link override sync_delay_x/Constant3: equ=P=C
  fft_stage_9 : fft_library/fft_stage_n  FFTSize=FFTSize  FFTStage=9  BitWidth=BitWidth  DelayBram=off  CoeffBram=on  MaxCoeffNum=MaxCoeffNum  quantization=Truncate  overflow=Wrap  add_latency=add_latency  mult_latency=mult_latency  bram_latency=bram_latency
      link override sync_delay_x/Constant: equ=P=C
      link override sync_delay_x/Constant1: equ=P=C
      link override sync_delay_x/Constant2: equ=P=C
      link override sync_delay_x/Constant3: equ=P=C
  out1 : Outport
  out2 : Outport  Port=2
  of : Outport  Port=3
  sync_out : Outport  Port=4
  wires:
  fft_stage_2/1(out1) -> fft_stage_3/1
  fft_stage_2/2(out2) -> fft_stage_3/2
  fft_stage_2/3(of) -> fft_stage_3/3
  fft_stage_2/4(sync_out) -> fft_stage_3/4
  shift/1 -> fft_stage_3/5, fft_stage_4/5, fft_stage_5/5, fft_stage_6/5, fft_stage_7/5, fft_stage_8/5, fft_stage_9/5, fft_stage_10/5, fft_stage_11/5, fft_stage_12/5, fft_stage_13/5, fft_stage_14/5, fft_stage_1/4(shift), fft_stage_2/5(shift)
  fft_stage_3/1 -> fft_stage_4/1
  fft_stage_3/2 -> fft_stage_4/2
  fft_stage_3/3 -> fft_stage_4/3
  fft_stage_3/4 -> fft_stage_4/4
  fft_stage_4/1 -> fft_stage_5/1
  fft_stage_4/2 -> fft_stage_5/2
  fft_stage_4/3 -> fft_stage_5/3
  fft_stage_4/4 -> fft_stage_5/4
  fft_stage_5/1 -> fft_stage_6/1
  fft_stage_5/2 -> fft_stage_6/2
  fft_stage_5/3 -> fft_stage_6/3
  fft_stage_5/4 -> fft_stage_6/4
  fft_stage_6/1 -> fft_stage_7/1
  fft_stage_6/2 -> fft_stage_7/2
  fft_stage_6/3 -> fft_stage_7/3
  fft_stage_6/4 -> fft_stage_7/4
  fft_stage_7/1 -> fft_stage_8/1
  fft_stage_7/2 -> fft_stage_8/2
  fft_stage_7/3 -> fft_stage_8/3
  fft_stage_7/4 -> fft_stage_8/4
  fft_stage_8/1 -> fft_stage_9/1
  fft_stage_8/2 -> fft_stage_9/2
  fft_stage_8/3 -> fft_stage_9/3
  fft_stage_8/4 -> fft_stage_9/4
  fft_stage_9/1 -> fft_stage_10/1
  fft_stage_9/2 -> fft_stage_10/2
  fft_stage_9/3 -> fft_stage_10/3
  fft_stage_9/4 -> fft_stage_10/4
  fft_stage_10/1 -> fft_stage_11/1
  fft_stage_10/2 -> fft_stage_11/2
  fft_stage_10/3 -> fft_stage_11/3
  fft_stage_10/4 -> fft_stage_11/4
  fft_stage_11/1 -> fft_stage_12/1
  fft_stage_11/2 -> fft_stage_12/2
  fft_stage_11/3 -> fft_stage_12/3
  fft_stage_11/4 -> fft_stage_12/4
  fft_stage_12/1 -> fft_stage_13/1
  fft_stage_12/2 -> fft_stage_13/2
  fft_stage_12/3 -> fft_stage_13/3
  fft_stage_12/4 -> fft_stage_13/4
  fft_stage_13/1 -> fft_stage_14/1
  fft_stage_13/2 -> fft_stage_14/2
  fft_stage_13/3 -> fft_stage_14/3
  fft_stage_13/4 -> fft_stage_14/4
  pol1/1 -> fft_stage_1/1(in1)
  pol2/1 -> fft_stage_1/2(in2)
  sync/1 -> fft_stage_1/3(sync)
  fft_stage_1/1(out1) -> fft_stage_2/1(in1)
  fft_stage_1/2(out2) -> fft_stage_2/2(in2)
  fft_stage_1/3(of) -> fft_stage_2/3(of_in)
  fft_stage_1/4(sync_out) -> fft_stage_2/4(sync)
  fft_stage_14/1 -> out1/1
  fft_stage_14/2 -> out2/1
  fft_stage_14/3 -> of/1
  fft_stage_14/4 -> sync_out/1

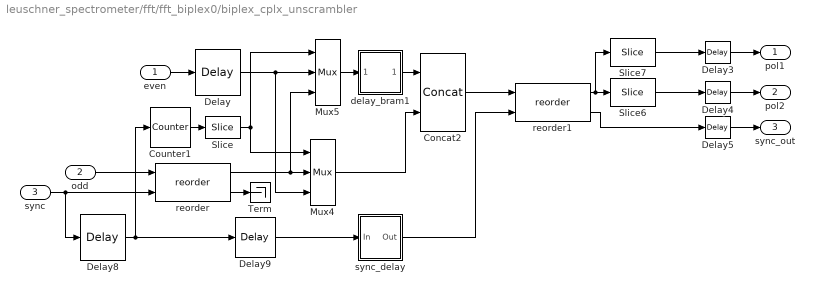
== system leuschner_spectrometer/fft/fft_biplex0/biplex_cplx_unscrambler ==
  even : Inport  Port=1  LatchInput=off
  odd : Inport  Port=2  LatchInput=off
  sync : Inport  Port=3  LatchInput=off
  Concat2 : xbsIndex_r3/Concat  num_inputs=2  explicit_period=off  period=1  dbl_ovrd=off
  Counter1 : xbsIndex_r3/Counter  cnt_type=Free Running  n_bits=FFTSize  bin_pt=0  arith_type=Unsigned  start_count=0  cnt_to=Inf  cnt_by_val=1  operation=Up  explicit_period=off  period=1  load_pin=off  rst=on  en=off  dbl_ovrd=off  show_param=off  use_rpm=off  gen_core=on
      settings: xl_area=[0, 0, 0, 0, 0, 0, 0]
  Delay : xbsIndex_r3/Delay  latency=bram_latency + 3  reg_retiming=off  explicit_period=off  period=1  en=off  accept_only_valid=off  init_zero=on  dbl_ovrd=off  show_param=off
      settings: xl_area=[0, 0, 0, 0, 0, 0, 0]
  Delay{3..5,9} (4 alike) : xbsIndex_r3/Delay  latency=1  reg_retiming=off  explicit_period=off  period=1  en=off  accept_only_valid=off  init_zero=on  dbl_ovrd=off  show_param=off
      settings: xl_area=[0, 0, 0, 0, 0, 0, 0]
  Delay8 : xbsIndex_r3/Delay  latency=bram_latency + 3  reg_retiming=off  explicit_period=off  period=1  en=off  accept_only_valid=off  init_zero=on  dbl_ovrd=off  show_param=off
      settings: xl_area=[0, 0, 0, 0, 0, 0, 0]
  Mux4 : xbsIndex_r3/Mux  inputs=2  precision=Full  arith_type="Signed  (2's comp)"  n_bits=8  bin_pt=2  quantization=Truncate  overflow=Wrap  latency=1  explicit_period=off  period=1  en=off  dbl_ovrd=off  show_param=off  mux_type=off  use_rpm=off  gen_core=on
      settings: xl_area=[0, 0, 0, 0, 0, 0, 0]
  Mux5 : xbsIndex_r3/Mux  inputs=2  precision=Full  arith_type="Signed  (2's comp)"  n_bits=8  bin_pt=2  quantization=Truncate  overflow=Wrap  latency=1  explicit_period=off  period=1  en=off  dbl_ovrd=off  show_param=off  mux_type=off  use_rpm=off  gen_core=on
      settings: xl_area=[0, 0, 0, 0, 0, 0, 0]
  Slice : xbsIndex_r3/Slice  mode=Upper Bit Location + Width  nbits=1  bit1=0  base1=MSB of Input  bit0=0  base0=LSB of Input  boolean_output=off  explicit_period=off  period=1  dbl_ovrd=off
  Slice6 : xbsIndex_r3/Slice  mode=Lower Bit Location + Width  nbits=2*BitWidth  bit1=-1  base1=MSB of Input  bit0=0  base0=LSB of Input  boolean_output=off  explicit_period=off  period=1  dbl_ovrd=off
  Slice7 : xbsIndex_r3/Slice  mode=Upper Bit Location + Width  nbits=2*BitWidth  bit1=0  base1=MSB of Input  bit0=0  base0=LSB of Input  boolean_output=off  explicit_period=off  period=1  dbl_ovrd=off
  Term : Terminator
  delay_bram1 : Subsystem  mask(delay_bram){DelayLen=2^(FFTSize-1), bram_latency=bram_latency}
      mask prompts: DelayLen "Delay By:"; bram_latency "BRAM Latency"
      mask init:
      | if (DelayLen <= bram_latency)
      | 	error('delay value must be greater than BRAM Latency');
      | end
      | BitWidth = max(ceil(log2(DelayLen)), 2);
      mask Display: fprintf('Z^-%d', DelayLen)
  reorder : fft_library/reorder  n_bits=FFTSize - 1  bit_reverse=off  ping_pong=off  bram_latency=bram_latency
      link override Constant: equ=P=C
      link override sync_delay/Constant: equ=P=C
      link override sync_delay/Constant1: equ=P=C
      link override sync_delay/Constant2: equ=P=C
      link override sync_delay/Constant3: equ=P=C
  reorder1 : fft_library/reorder  n_bits=FFTSize - 1  bit_reverse=on  ping_pong=off  bram_latency=bram_latency
      link override Constant: equ=P=C
      link override sync_delay/Constant: equ=P=C
      link override sync_delay/Constant1: equ=P=C
      link override sync_delay/Constant2: equ=P=C
      link override sync_delay/Constant3: equ=P=C
  sync_delay : Subsystem  mask{DelayLen=2^(FFTSize-1)}
      mask prompts: DelayLen "Delay Length:"
      mask init:
      | BitWidth = max(2, ceil(log2(DelayLen+1)));
      | UseCounter = 1;
      | if DelayLen == 0,
      | 	UseCounter = 0;
      | end
      mask Display: fprintf('Z^-%d', DelayLen)
  pol1 : Outport
  pol2 : Outport  Port=2
  sync_out : Outport  Port=3
  wires:
  sync_delay/1(Out) -> reorder1/2
  delay_bram1/1(Out1) -> Concat2/1
  even/1 -> Delay/1
  odd/1 -> reorder/1
  sync/1 -> reorder/2, Delay8/1
  reorder/2 -> Term/1
  Delay8/1 -> Counter1/1, Delay9/1
  Delay9/1 -> sync_delay/1(In)
  Counter1/1 -> Slice/1
  Mux4/1 -> Concat2/2
  Mux5/1 -> delay_bram1/1(In1)
  reorder/1 -> Mux5/3, Mux4/2
  Delay/1 -> Mux4/3, Mux5/2
  Slice/1 -> Mux4/1, Mux5/1
  Concat2/1 -> reorder1/1
  reorder1/1 -> Slice6/1, Slice7/1
  Slice7/1 -> Delay3/1
  Slice6/1 -> Delay4/1
  reorder1/2 -> Delay5/1
  Delay3/1 -> pol1/1
  Delay4/1 -> pol2/1
  Delay5/1 -> sync_out/1

== system leuschner_spectrometer/power/vacc_64bit0/delay1 ==
  In1 : Inport  Port=1  LatchInput=off
  delay_bram : casper_library/Delays/delay_bram  DelayLen=2^13-4  bram_latency=2
  Out1 : Outport
  wires:
  In1/1 -> delay_bram/1
  delay_bram/1 -> Out1/1

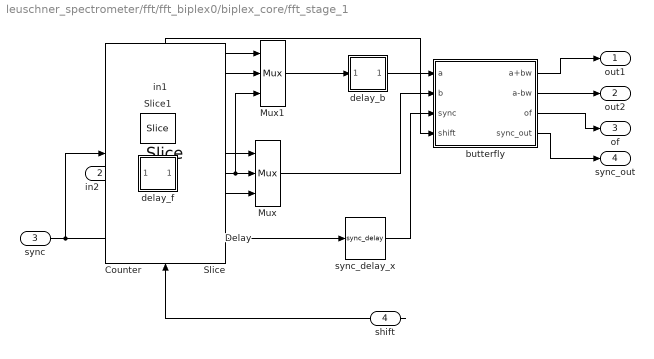
== system leuschner_spectrometer/fft/fft_biplex0/biplex_core/fft_stage_1 ==
  in1 : Inport  Port=1  LatchInput=off
  in2 : Inport  Port=2  LatchInput=off
  sync : Inport  Port=3  LatchInput=off
  shift : Inport  Port=4  LatchInput=off
  Counter : xbsIndex_r3/Counter  cnt_type=Free Running  n_bits=FFTSize-FFTStage+1  bin_pt=0  arith_type=Unsigned  start_count=0  cnt_to=Inf  cnt_by_val=1  operation=Up  explicit_period=off  period=1  load_pin=off  rst=on  en=off  dbl_ovrd=off  show_param=off  use_rpm=off  gen_core=on
      settings: xl_area=[0, 0, 0, 0, 0, 0, 0]
  Delay : xbsIndex_r3/Delay  latency=1  reg_retiming=off  explicit_period=off  period=1  en=off  accept_only_valid=off  init_zero=on  dbl_ovrd=off  show_param=off
      settings: xl_area=[0, 0, 0, 0, 0, 0, 0]
  Mux : xbsIndex_r3/Mux  inputs=2  precision=Full  arith_type="Signed  (2's comp)"  n_bits=8  bin_pt=2  quantization=Truncate  overflow=Wrap  latency=1  explicit_period=off  period=1  en=off  dbl_ovrd=off  show_param=off  mux_type=off  use_rpm=off  gen_core=on
      settings: xl_area=[0, 0, 0, 0, 0, 0, 0]
  Mux1 : xbsIndex_r3/Mux  inputs=2  precision=Full  arith_type="Signed  (2's comp)"  n_bits=8  bin_pt=2  quantization=Truncate  overflow=Wrap  latency=1  explicit_period=off  period=1  en=off  dbl_ovrd=off  show_param=off  mux_type=off  use_rpm=off  gen_core=on
      settings: xl_area=[0, 0, 0, 0, 0, 0, 0]
  Slice : xbsIndex_r3/Slice  Orientation=up  mode=Lower Bit Location + Width  nbits=1  bit1=-(FFTStage - 1)  base1=MSB of Input  bit0=FFTStage - 1  base0=LSB of Input  boolean_output=on  explicit_period=off  period=1  dbl_ovrd=off
  Slice1 : xbsIndex_r3/Slice  mode=Upper Bit Location + Width  nbits=1  bit1=0  base1=MSB of Input  bit0=0  base0=LSB of Input  boolean_output=off  explicit_period=off  period=1  dbl_ovrd=off
  butterfly : Subsystem
  delay_b : Subsystem  BlockChoice=delay_bram
      link override delay_bram: DelayLen=2^(FFTSize-FFTStage)  bram_latency=bram_latency
      link override delay_bram/Constant2: equ=P=C
      link override delay_slr: DelayLen=2^(FFTSize-FFTStage)
      settings: AttributesFormatString=%<BlockChoice>  TemplateBlock=delay_lib/delay  MemberBlocks=delay_bram,delay_slr
  delay_f : Subsystem  BlockChoice=delay_bram
      link override delay_bram: DelayLen=2^(FFTSize-FFTStage)  bram_latency=bram_latency
      link override delay_bram/Constant2: equ=P=C
      link override delay_slr: DelayLen=2^(FFTSize-FFTStage)
      settings: AttributesFormatString=%<BlockChoice>  TemplateBlock=delay_lib/delay  MemberBlocks=delay_bram,delay_slr
  sync_delay_x : fft_library/sync_delay  DelayLen=2^(FFTSize - FFTStage)
      link override Constant: equ=P=C
      link override Constant1: equ=P=C
      link override Constant2: equ=P=C
      link override Constant3: equ=P=C
  out1 : Outport
  out2 : Outport  Port=2
  of : Outport  Port=3
  sync_out : Outport  Port=4
  wires:
  butterfly/4(sync_out) -> sync_out/1
  butterfly/1(a+bw) -> out1/1
  butterfly/2(a-bw) -> out2/1
  butterfly/3(of) -> of/1
  Slice/1 -> butterfly/4(shift)
  sync_delay_x/1 -> butterfly/3(sync)
  delay_b/1(Out1) -> butterfly/1(a)
  in2/1 -> delay_f/1(In1)
  Slice1/1 -> Mux1/1, Mux/1
  in1/1 -> Mux1/2, Mux/3
  delay_f/1(Out1) -> Mux/2, Mux1/3
  Mux1/1 -> delay_b/1(In1)
  Mux/1 -> butterfly/2(b)
  Counter/1 -> Slice1/1
  sync/1 -> Delay/1, Counter/1
  Delay/1 -> sync_delay_x/1
  shift/1 -> Slice/1
